simulink model "feedback_template"  (R2023b)
settings: Solver=VariableStepAuto  StartTime=0.0  StopTime=10.0  RelTol=1e-3
values from neighbouring files (symbols this model uses):
  A_ob = A - L*C    [main_feedback_lin.m]
  B_ob = [ B - L*D, L]    [main_feedback_lin.m]
  C_ob = eye(n)    [main_feedback_lin.m]
  D_ob = zeros(n, m+p)    [main_feedback_lin.m]
  Upper_bound_V = 23    [PI_comparison.m]    (also in main_feedback_lin.m)
undefined symbols (not defined in the file or in its folder): HIL, Kb, offset_corrente_volt, offset_posizione_volt, x1_eq0, x2_eq0, x3_eq0
libraries: quarc_library x4, simulink x1
settings Model: Creator=Pronto all'uso  LastModifiedBy=lollo
settings SolverCC: AlgebraicLoopSolver=TrustRegion

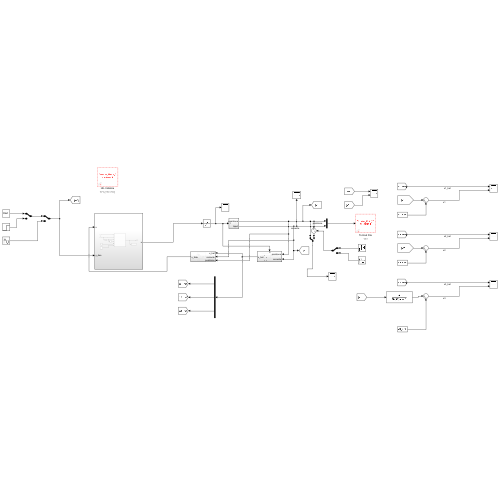
[thumbnail: Simulink's stored preview of the top-level diagram]
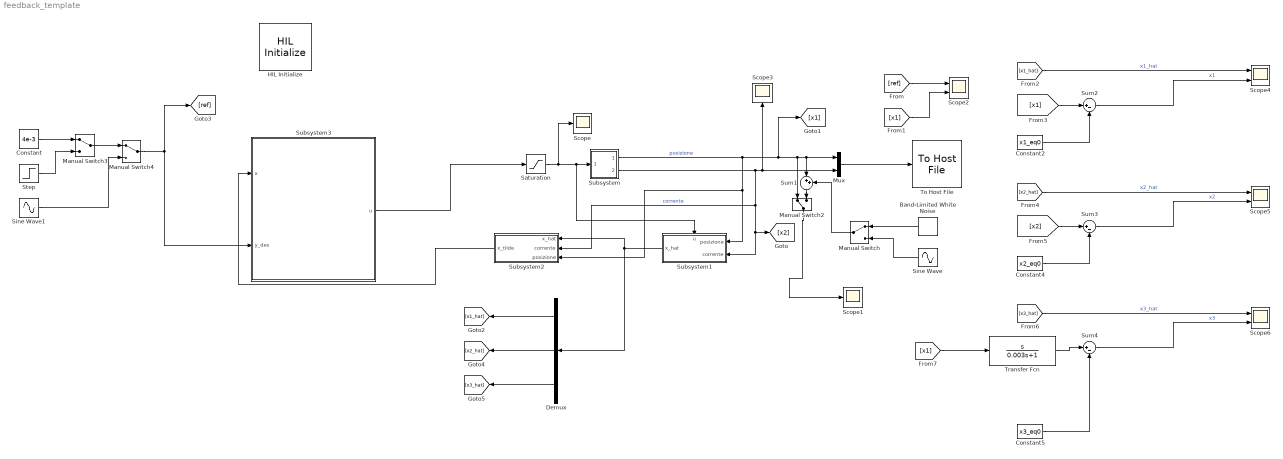
== system feedback_template ==
  Band-Limited White Noise : simulink/Sources/Band-Limited White Noise  Cov=[8.9934e-11*0.002]  Ts=0.002  seed=[23341]
  Constant : Constant  Value=4e-3
  Constant2 : Constant  Value=x1_eq0
  Constant4 : Constant  Value=x2_eq0
  Constant5 : Constant  Value=x3_eq0
  Demux : Demux  Outputs=3
  HIL Initialize : quarc_library/Data Acquisition/Generic/Configuration/HIL Initialize  Priority=-99  object_name=HIL-1  board_type=q2_usb  board_number=0  board_options=d0=digital;d1=digital;led=auto;update_rate=normal;decimation=1  exclusive=off  active=off  hardware_clocks=[0]  clock_modes=[]  initial_clock_frequencies=[]  set_clock_params_at_start=off  set_clock_params_at_switch_in=off  set_clock_frequencies_at_start=off  set_clock_frequencies_at_switch_in=off  analog_input_channels=[0:1]  analog_input_configurations=[]  analog_input_maximums=10  analog_input_minimums=-10  set_analog_input_params_at_start=on  set_analog_input_params_at_switch_in=off  analog_output_channels=[0:1]  analog_output_maximums=10  analog_output_minimums=-10  initial_analog_outputs=[0]  final_analog_outputs=[0]  watchdog_analog_outputs=0  set_analog_output_params_at_start=on  set_analog_output_params_at_switch_in=off  set_analog_outputs_at_start=on  set_analog_outputs_at_switch_in=off  set_analog_outputs_at_terminate=on  set_analog_outputs_at_switch_out=off  set_analog_outputs_on_watchdog=off  digital_input_channels=[]  digital_output_channels=[]  digital_output_configuration=[]  initial_digital_outputs=[1]  final_digital_outputs=[1]  watchdog_digital_outputs=[1]  set_digital_output_params_at_start=off  set_digital_output_params_at_switch_in=off  set_digital_outputs_at_start=on  set_digital_outputs_at_switch_in=off  set_digital_outputs_at_terminate=on  set_digital_outputs_at_switch_out=off  set_digital_outputs_on_watchdog=off  encoder_channels=[0:1]  quadrature=[4]  encoder_filter_frequency=[]  initial_encoder_counts=[0]  set_encoder_params_at_start=on  set_encoder_params_at_switch_in=off  set_encoder_counts_at_start=on  set_encoder_counts_at_switch_in=off  pwm_channels=[]  pwm_modes=[0]  pwm_frequency=1/0.020  pwm_configuration=[]  pwm_alignment=[]  pwm_polarity=[]  pwm_leading_deadband=[]  pwm_trailing_deadband=[]  initial_pwm_outputs=[0]  final_pwm_outputs=[0]  watchdog_pwm_outputs=[0]  set_pwm_params_at_start=on  set_pwm_params_at_switch_in=off  set_pwm_outputs_at_start=on  set_pwm_outputs_at_switch_in=off  set_pwm_outputs_at_terminate=on  set_pwm_outputs_at_switch_out=off  set_pwm_outputs_on_watchdog=off  other_output_channels=[]  initial_other_outputs=[]  final_other_outputs=[]  watchdog_other_outputs=[]  set_other_outputs_at_start=off  set_other_outputs_at_switch_in=off  set_other_outputs_at_terminate=off  set_other_outputs_at_switch_out=off  set_other_outputs_on_watchdog=off
  Manual Switch{,2..4} (4 alike) : ManualSwitch
  Mux : Mux  Inputs=2
  Saturation : Saturate  UpperLimit=Upper_bound_V  LowerLimit=0
  Scope : Scope
  Scope1 : Scope
  Scope{2,4..6} (4 alike) : Scope  NumInputPorts=2
  Scope3 : Scope
  Sine Wave : Sin  SampleTime=0
  Sine Wave1 : Sin  SampleTime=0
  Step : Step  Time=2  After=0.003  SampleTime=0
  Subsystem : Subsystem
  Subsystem1 : Subsystem
      settings: PortSchema="{\"entries\":[{\"content\":{\"sides\":[{\"content\":{\"connectorIds\":[\"In1\",\"In2\"]},\"type\":\"ConnectorPlacement.EquallySpacedRectSide\",\"uuid\":\"e1f8050f-b2dc-4f8d-845a-8e8b9880ba58\"},{\"content\":{\"connectorIds\":[\"Out1\"],\"side\":\"RIGHT\"},\"type\":\"ConnectorPlacement.EquallySpacedRectSide\",\"uuid\":\"2dff5a5a-bb20-48d2-8c33-afdcadaef98a\"},{\"content\":{\"connectorIds\":[\"In3\"],\"side\":\"TOP\"},\"type\":\"ConnectorPlacement.EquallySpacedRectSide\",\"uuid\":\"a11ee514-1b89-428e-a461-d5594e2b13e4\"}]},\"type\":\"ConnectorPlacement.EquallySpacedConnector\",\"uuid\":\"4c472648-3e9d-49b6-afa0-83f39b537fb6\"}],\"packageUris\":[\"http://schema.mathworks.com/mf0/Connector/R2020b\"],\"version\":\"1.0\"}"
  Subsystem2 : Subsystem
  Subsystem3 : Subsystem
  Sum1 : Sum  Inputs=|++
  Sum2 : Sum  Inputs=|+-
  Sum3 : Sum  Inputs=|+-
  Sum4 : Sum  Inputs=|+-
  To Host File : quarc_library/Sinks/To Host/To Host File  file_name=data_%{date}_%{time}.mat  variable_name=data_%{date}_%{time}  decimation=1  sample_time=-1  file_format=MAT-file v.5  options=No header or footer  append=off  final_file_name=data_06-May-2025_18-58-45.mat  bitrate=2000000
  Transfer Fcn : TransferFcn  Numerator=[1 0]  Denominator=[0.003 1]
  wires:
  [x1] -> Scope2/2
  Mux/1 -> To Host File/1
  Manual Switch/1 -> Sum1/2
  Constant/1 -> Manual Switch3/1
  Sine Wave/1 -> Manual Switch/2
  Band-Limited White Noise/1 -> Manual Switch/1
  Manual Switch3/1 -> Manual Switch4/1
  Subsystem/2(Input) -> Subsystem2/2(corrente), [x2], Subsystem1/2(corrente), Scope3/1, Mux/2  "corrente"
  Manual Switch2/1 -> Scope1/1
  Subsystem3/1(u) -> Saturation/1
  [ref] -> Scope2/1
  Step/1 -> Manual Switch3/2
  Sine Wave1/1 -> Manual Switch4/2
  Subsystem/1(posizione) -> [x1], Manual Switch2/1, Mux/1, Sum1/1, Subsystem2/3(posizione), Subsystem1/1(posizione)  "posizione"
  Sum1/1 -> Manual Switch2/2
  Manual Switch4/1 -> Subsystem3/2(y_des), [ref]
  Saturation/1 -> Scope/1, Subsystem1/3(u), Subsystem/1(In1)
  Subsystem1/1(x_hat) -> Subsystem2/1(x_hat), Demux/1
  Demux/2 -> [x2_hat]
  Demux/1 -> [x1_hat]
  Demux/3 -> [x3_hat]
  [x2_hat] -> Scope5/1  "x2_hat"
  Constant4/1 -> Sum3/2
  Sum4/1 -> Scope6/2  "x3"
  Sum3/1 -> Scope5/2  "x2"
  Constant5/1 -> Sum4/2
  [x1] -> Sum2/1
  [x3_hat] -> Scope6/1  "x3_hat"
  Transfer Fcn/1 -> Sum4/1
  Sum2/1 -> Scope4/2  "x1"
  [x1_hat] -> Scope4/1  "x1_hat"
  Constant2/1 -> Sum2/2
  [x2] -> Sum3/1
  Subsystem2/1(x_tilde) -> Subsystem3/1(x)
  [x1] -> Transfer Fcn/1

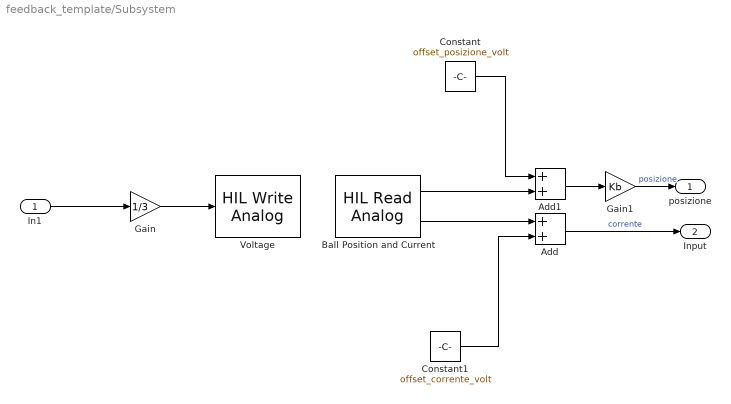
== system feedback_template/Subsystem ==
  In1 : Inport
  Add : Sum
  Add1 : Sum
  Ball Position and Current : quarc_library/Data Acquisition/Generic/Immediate I//O/HIL Read Analog  object_name=HIL-1  channels=[0:1]  sample_time=qc_get_step_size  active=on  vector_output=off
  Constant : Constant  Value=offset_posizione_volt
  Constant1 : Constant  Value=offset_corrente_volt
  Gain : Gain  Gain=1/3
  Gain1 : Gain  Gain=Kb
  Voltage : quarc_library/Data Acquisition/Generic/Immediate I//O/HIL Write Analog  object_name=HIL-1  channels=0  sample_time=-1  active=off  vector_input=off
  posizione : Outport
  Input : Outport  Port=2
  wires:
  Ball Position and Current/1 -> Add1/2
  In1/1 -> Gain/1
  Ball Position and Current/2 -> Add/1
  Gain/1 -> Voltage/1
  Gain1/1 -> posizione/1  "posizione"
  Add1/1 -> Gain1/1
  Add/1 -> Input/1  "corrente"
  Constant1/1 -> Add/2
  Constant/1 -> Add1/1

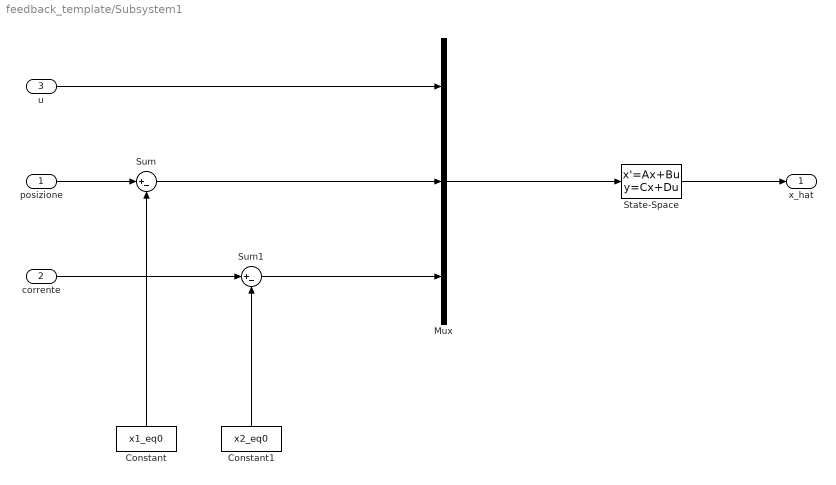
== system feedback_template/Subsystem1 ==
  posizione : Inport
  corrente : Inport  Port=2
  u : Inport  Port=3
  Constant : Constant  Value=x1_eq0
  Constant1 : Constant  Value=x2_eq0
  Mux : Mux  Inputs=3
  State-Space : StateSpace  A=A_ob  B=B_ob  C=C_ob  D=D_ob  InitialCondition=[-x1_eq0, -x2_eq0, 0]
  Sum : Sum  Inputs=|+-
  Sum1 : Sum  Inputs=|+-
  x_hat : Outport
  wires:
  posizione/1 -> Sum/1
  Constant/1 -> Sum/2
  Constant1/1 -> Sum1/2
  corrente/1 -> Sum1/1
  u/1 -> Mux/1
  Sum/1 -> Mux/2
  Sum1/1 -> Mux/3
  State-Space/1 -> x_hat/1
  Mux/1 -> State-Space/1

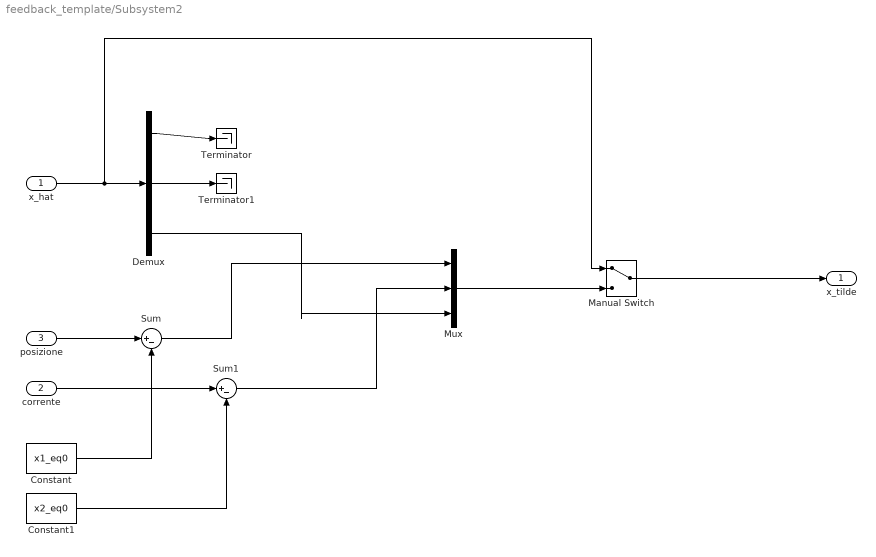
== system feedback_template/Subsystem2 ==
  x_hat : Inport
  corrente : Inport  Port=2
  posizione : Inport  Port=3
  Constant : Constant  Value=x1_eq0
  Constant1 : Constant  Value=x2_eq0
  Demux : Demux  Outputs=3
  Manual Switch : ManualSwitch
  Mux : Mux  Inputs=3
  Sum : Sum  Inputs=|+-
  Sum1 : Sum  Inputs=|+-
  Terminator : Terminator
  Terminator1 : Terminator
  x_tilde : Outport
  wires:
  x_hat/1 -> Manual Switch/1, Demux/1
  Manual Switch/1 -> x_tilde/1
  Demux/1 -> Terminator/1
  Demux/2 -> Terminator1/1
  Mux/1 -> Manual Switch/2
  Demux/3 -> Mux/3
  posizione/1 -> Sum/1
  corrente/1 -> Sum1/1
  Sum/1 -> Mux/1
  Sum1/1 -> Mux/2
  Constant/1 -> Sum/2
  Constant1/1 -> Sum1/2

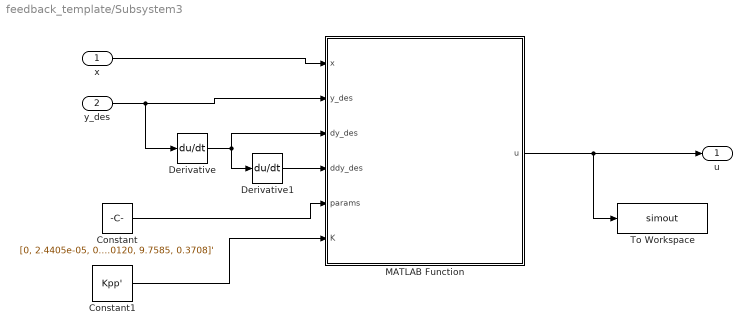
== system feedback_template/Subsystem3 ==
  x : Inport
  y_des : Inport  Port=2
  Constant : Constant  Value=[0, 2.4405e-05, 0.0657, 0.0120, 9.7585, 0.3708]'
  Constant1 : Constant  Value=Kpp'
  Derivative : Derivative
  Derivative1 : Derivative
  MATLAB Function : MATLAB Function  TreatAsAtomicUnit=on
  To Workspace : ToWorkspace  VariableName=simout  SaveFormat=Timeseries  SampleTime=-1
  u : Outport
  wires:
  y_des/1 -> Derivative/1, MATLAB Function/2(y_des)
  x/1 -> MATLAB Function/1(x)
  MATLAB Function/1(u) -> To Workspace/1, u/1
  Derivative/1 -> Derivative1/1, MATLAB Function/3(dy_des)
  Constant/1 -> MATLAB Function/5(params)
  Derivative1/1 -> MATLAB Function/4(ddy_des)
  Constant1/1 -> MATLAB Function/6(K)

== matlab function feedback_template/Subsystem3/MATLAB Function ==
  data: x input; u output; y_des input; dy_des input; ddy_des input; params input; K input
function u = feedback_linearization_control(x, y_des, dy_des, ddy_des, params, K)
    % Estrai parametri
    k_aero = params(1);
    k_mag  = params(2);
    m      = params(3);
    y0     = params(4);
    Rtot   = params(5);
    Lc     = params(6);
    g      = 9.81;

    % Stati
    x1 = x(1); % posizione
    x2 = x(2); % corrente
    x3 = x(3); % velocità

    % Derivate
    denom = (y0 - x1);
    if denom <= 0
        error('Denominatore nullo o negativo: instabilità elettromagnetica');
    end

    % Calcola seconda derivata (accelerazione)
    xdot3 = (k_aero/m)*x3 + (k_mag/m)*(x2 / denom)^2 - g;

    % Calcola derivata di corrente x2 (richiede input u)
    % da: dx2 = -(Rtot/Lc)*x2 + (1/Lc)*u;
    % => u comparirà nella terza derivata

    % Calcolo della terza derivata (solo parte non u)
    dBdx1 = (2 * k_mag * x2^2) / (m * denom^3);
    dBdx2 = (4 * k_mag * x2) / (m * denom^2);
    dBdx3 = (k_aero/m);

    % Parte non lineare alpha(x)
    alpha = dBdx1 * x3 + dBdx2 * (-(Rtot/Lc)*x2) + dBdx3 * xdot3;

    % Parte moltiplicativa davanti a u (beta(x))
    beta = dBdx2 * (1/Lc);

    % Guadagni desiderati (dati da specifica: esempio polo a - 2, -2, -3)
    
    e = x1 - y_des;
    de = x3 - dy_des;
    dde = xdot3 - ddy_des;
    assignin('base', 'e', e)
    assignin('base', 'ed', de)
    assignin('base', 'edd', dde)

    v = -K' * [e; de; dde];

    % Controllo finale
    u = (1/beta) * (v - alpha);
end
